simulink model "compensation_simul"  (R2019a)
settings: Solver=VariableStepAuto  StartTime=0.0  StopTime=10.0  RelTol=1e-3
values from neighbouring files (symbols this model uses):
  kc = (Tc/(k*Kp_id))*p1*p2    [Compensator.m]
  Kp_id = 10/50    (= 0.2)    [Compensator.m]
  T = 0.2024    [Compensator.m]
  Tc = -1/(p1+p2)    [Compensator.m]
settings Model: Creator=xde12  LastModifiedBy=xde12

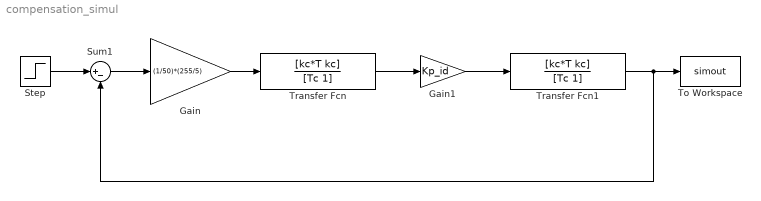
== system compensation_simul ==
  Gain : Gain  Gain=(1/50)*(255/5)
  Gain1 : Gain  Gain=Kp_id
  Step : Step  SampleTime=0
  Sum1 : Sum  Inputs=|+-
  To Workspace : ToWorkspace  VariableName=simout  SampleTime=-1
      settings: Save2DSignal=2-D array (concatenate along first dimension)
  Transfer Fcn : TransferFcn  Numerator=[kc*T kc]  Denominator=[Tc 1]
  Transfer Fcn1 : TransferFcn  Numerator=[kc*T kc]  Denominator=[Tc 1]
  wires:
  Gain/1 -> Transfer Fcn/1
  Transfer Fcn/1 -> Gain1/1
  Sum1/1 -> Gain/1
  Gain1/1 -> Transfer Fcn1/1
  Transfer Fcn1/1 -> To Workspace/1, Sum1/2
  Step/1 -> Sum1/1
